simulink model "biplex_core_plan"  (Simulink 7.6)
settings: Solver=ode45  StartTime=0.0  StopTime=10.0  RelTol=1e-3
libraries: xbsIndex_r4 x121, monroe_library x13
settings Model: Creator=Ryan  LastModifiedBy=Ryan

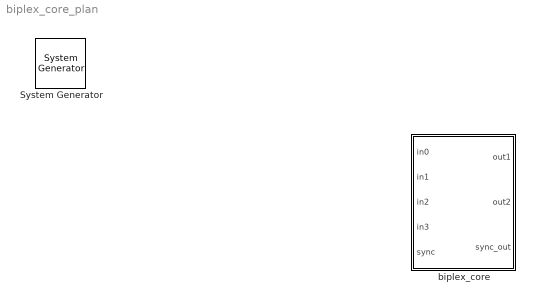
== system biplex_core_plan ==
  " System Generator" : xbsIndex_r4/ System Generator  Tag=genX  SystemSampleTime=-1  xilinxfamily=Virtex6  part=xc6vsx315t  speed=-3  package=ff1156  synthesis_tool=XST  clock_wrapper=Clock Enables  directory=./netlist  testbench=off  simulink_period=1  sysclk_period=10  dcm_input_clock_period=10  incr_netlist=off  trim_vbits=Everywhere in SubSystem  dbl_ovrd=According to Block Masks  core_generation=According to Block Masks  run_coregen=off  deprecated_control=off  eval_field=0  block_type=sysgen
  biplex_core : Subsystem
  wires:
  ? -> biplex_core/5(sync)

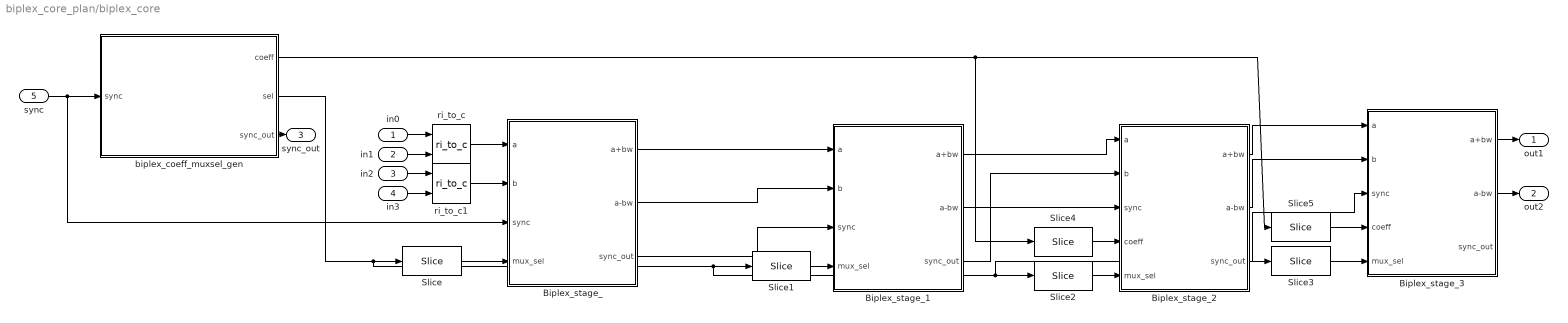
== system biplex_core_plan/biplex_core ==
  in0 : Inport
  in1 : Inport  Port=2
  in2 : Inport  Port=3
  in3 : Inport  Port=4
  sync : Inport  Port=5
  Biplex_stage_ : Subsystem  mask{FFTSize=4, FFTStage=1, input_bit_width=18, coeff_bit_width=18, output_bit_width=18, delays_bram=1, bram_latency=2, shift=0, delay_arr=[0,1,0]}
      mask prompts: FFTSize "FFT Size"; FFTStage "FFT Stage"; input_bit_width "Input Bit Width"; coeff_bit_width "Coefficient Bit Width"; output_bit_width "Output Bit Width"; delays_bram "Delays in BRAM"; bram_latency "BRAM latency"; shift "Downshift in this stage? (0 or 1)"; delay_arr "In-Stage Delay Array"
      mask init:
      | config.source=str2func('biplex_stage_n_draw');
      | config.toplevel=gcb;
      | config.debug=0;
      | config.depend={'biplex_stage_n_draw.m'};
      | xBlock(config,{FFTSize, FFTStage, input_bit_width, coeff_bit_width, output_bit_width, delays_bram, bram_latency, shift, delay_arr});
  Biplex_stage_1 : Subsystem  mask{FFTSize=4, FFTStage=2, input_bit_width=18, coeff_bit_width=18, output_bit_width=18, delays_bram=1, bram_latency=2, shift=0, delay_arr=[0,1,0]}
      mask prompts: FFTSize "FFT Size"; FFTStage "FFT Stage"; input_bit_width "Input Bit Width"; coeff_bit_width "Coefficient Bit Width"; output_bit_width "Output Bit Width"; delays_bram "Delays in BRAM"; bram_latency "BRAM latency"; shift "Downshift in this stage? (0 or 1)"; delay_arr "In-Stage Delay Array"
      mask init: same as biplex_core_plan/biplex_core/Biplex_stage_
  Biplex_stage_2 : Subsystem  mask{FFTSize=4, FFTStage=3, input_bit_width=18, coeff_bit_width=18, output_bit_width=18, delays_bram=1, bram_latency=2, shift=0, delay_arr=[0,1,0]}
      mask prompts: FFTSize "FFT Size"; FFTStage "FFT Stage"; input_bit_width "Input Bit Width"; coeff_bit_width "Coefficient Bit Width"; output_bit_width "Output Bit Width"; delays_bram "Delays in BRAM"; bram_latency "BRAM latency"; shift "Downshift in this stage? (0 or 1)"; delay_arr "In-Stage Delay Array"
      mask init: same as biplex_core_plan/biplex_core/Biplex_stage_
  Biplex_stage_3 : Subsystem  mask{FFTSize=4, FFTStage=4, input_bit_width=18, coeff_bit_width=18, output_bit_width=18, delays_bram=1, bram_latency=2, shift=0, delay_arr=[0,1,0]}
      mask prompts: FFTSize "FFT Size"; FFTStage "FFT Stage"; input_bit_width "Input Bit Width"; coeff_bit_width "Coefficient Bit Width"; output_bit_width "Output Bit Width"; delays_bram "Delays in BRAM"; bram_latency "BRAM latency"; shift "Downshift in this stage? (0 or 1)"; delay_arr "In-Stage Delay Array"
      mask init: same as biplex_core_plan/biplex_core/Biplex_stage_
  Slice : xbsIndex_r4/Slice  nbits=1  boolean_output=on  mode=Upper Bit Location + Width  bit1=0  base1=MSB of Input  bit0=0  base0=LSB of Input  dbl_ovrd=off  block_type=slice
  Slice1 : xbsIndex_r4/Slice  nbits=1  boolean_output=on  mode=Upper Bit Location + Width  bit1=-1  base1=MSB of Input  bit0=0  base0=LSB of Input  dbl_ovrd=off  block_type=slice
  Slice2 : xbsIndex_r4/Slice  nbits=1  boolean_output=on  mode=Upper Bit Location + Width  bit1=-2  base1=MSB of Input  bit0=0  base0=LSB of Input  dbl_ovrd=off  block_type=slice
  Slice3 : xbsIndex_r4/Slice  nbits=1  boolean_output=on  mode=Upper Bit Location + Width  bit1=-3  base1=MSB of Input  bit0=0  base0=LSB of Input  dbl_ovrd=off  block_type=slice
  Slice4 : xbsIndex_r4/Slice  nbits=36  boolean_output=off  mode=Upper Bit Location + Width  bit1=0  base1=MSB of Input  bit0=0  base0=LSB of Input  dbl_ovrd=off  block_type=slice
  Slice5 : xbsIndex_r4/Slice  nbits=36  boolean_output=off  mode=Upper Bit Location + Width  bit1=-36  base1=MSB of Input  bit0=0  base0=LSB of Input  dbl_ovrd=off  block_type=slice
  biplex_coeff_muxsel_gen : Subsystem  mask{FFTSize=4, bit_width=18, register_coeffs=0, optional_delay_arr=[[1,0,1]; [1,1,1];  [1,1,1];  [1,1,1]], stage_delay_arr=[3,6,6,6]}
      mask prompts: FFTSize "FFT Size"; bit_width "Coefficient Bit Width"; register_coeffs "Register Coeffs?"; optional_delay_arr "In-Stage Delay Array"; stage_delay_arr "Mandatory Stage Delay Array"
      mask init:
      | config.source=str2func('biplex_coeff_muxsel_gen_draw');
      | config.toplevel=gcb;
      | config.debug=0;
      | config.depend={'biplex_coeff_muxsel_gen_draw.m'};
      | xBlock(config,{FFTSize, bit_width, register_coeffs, optional_delay_arr, stage_delay_arr});
  ri_to_c : monroe_library/ri_to_c  SystemSampleTime=-1
  ri_to_c1 : monroe_library/ri_to_c  SystemSampleTime=-1
  out1 : Outport
  out2 : Outport  Port=2
  sync_out : Outport  Port=3
  wires:
  ri_to_c/1 -> Biplex_stage_/1(a)
  ri_to_c1/1 -> Biplex_stage_/2(b)
  Biplex_stage_/3(sync_out) -> Biplex_stage_1/3(sync)
  Biplex_stage_/2(a-bw) -> Biplex_stage_1/2(b)
  Biplex_stage_/1(a+bw) -> Biplex_stage_1/1(a)
  Biplex_stage_1/1(a+bw) -> Biplex_stage_2/1(a)
  Biplex_stage_1/2(a-bw) -> Biplex_stage_2/2(b)
  Biplex_stage_1/3(sync_out) -> Biplex_stage_2/3(sync)
  Biplex_stage_2/1(a+bw) -> Biplex_stage_3/1(a)
  Biplex_stage_2/2(a-bw) -> Biplex_stage_3/2(b)
  Biplex_stage_2/3(sync_out) -> Biplex_stage_3/3(sync)
  biplex_coeff_muxsel_gen/2(sel) -> Slice/1, Slice1/1, Slice2/1, Slice3/1
  Slice/1 -> Biplex_stage_/4(mux_sel)
  Slice2/1 -> Biplex_stage_2/5(mux_sel)
  Slice1/1 -> Biplex_stage_1/4(mux_sel)
  Slice3/1 -> Biplex_stage_3/5(mux_sel)
  sync/1 -> biplex_coeff_muxsel_gen/1(sync), Biplex_stage_/3(sync)
  Slice5/1 -> Biplex_stage_3/4(coeff)
  biplex_coeff_muxsel_gen/1(coeff) -> Slice5/1, Slice4/1
  Slice4/1 -> Biplex_stage_2/4(coeff)
  in0/1 -> ri_to_c/1
  biplex_coeff_muxsel_gen/3(sync_out) -> sync_out/1
  Biplex_stage_3/1(a+bw) -> out1/1
  in1/1 -> ri_to_c/2
  in2/1 -> ri_to_c1/1
  in3/1 -> ri_to_c1/2
  Biplex_stage_3/2(a-bw) -> out2/1

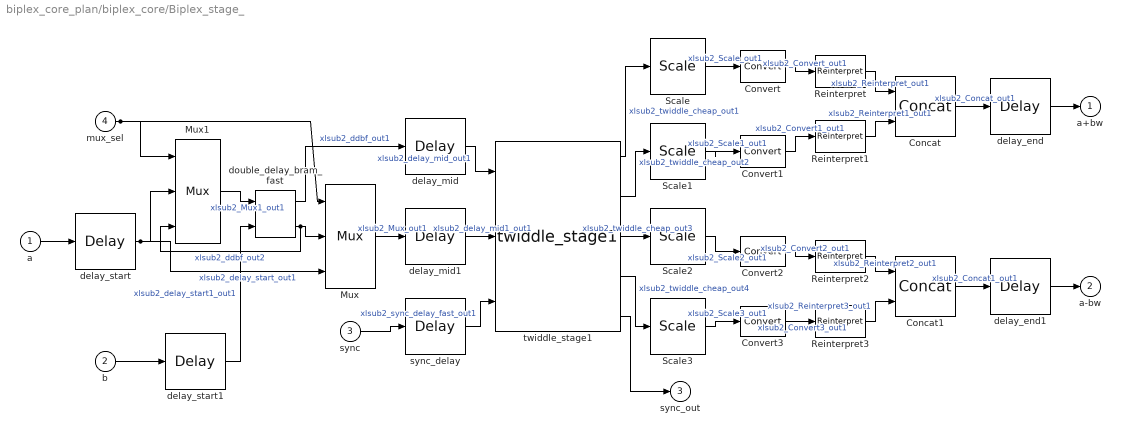
== system biplex_core_plan/biplex_core/Biplex_stage_ ==
  a : Inport
  b : Inport  Port=2
  sync : Inport  Port=3
  mux_sel : Inport  Port=4
  Concat : xbsIndex_r4/Concat  num_inputs=2  dbl_ovrd=off  block_type=concat
  Concat1 : xbsIndex_r4/Concat  num_inputs=2  dbl_ovrd=off  block_type=concat
  Convert{,1..3} (4 alike) : xbsIndex_r4/Convert  arith_type="Signed  (2's comp)"  n_bits=18  bin_pt=17  quantization=Truncate  overflow=Wrap  en=off  latency=0  dbl_ovrd=off  pipeline=off  block_type=convert
  Mux : xbsIndex_r4/Mux  inputs=2  en=off  latency=0  precision=Full  arith_type="Signed  (2's comp)"  n_bits=8  bin_pt=2  quantization=Truncate  overflow=Wrap  dbl_ovrd=off  block_type=mux
  Mux1 : xbsIndex_r4/Mux  inputs=2  en=off  latency=0  precision=Full  arith_type="Signed  (2's comp)"  n_bits=8  bin_pt=2  quantization=Truncate  overflow=Wrap  dbl_ovrd=off  block_type=mux
  Reinterpret{,1..3} (4 alike) : xbsIndex_r4/Reinterpret  force_arith_type=off  arith_type=Unsigned  force_bin_pt=off  bin_pt=0  block_type=reinterpret
      settings: infoedit="Changes signal type without altering the binary representation.   You can changed the signal between signed and unsigned, and relocate the binary point.<br><br>Hardware notes: In hardware this block costs nothing.<br><br>Example:  Suppose the input is 6 bits wide, signed, with 2 fractional bits, and the output is forced to unsigned with 0 fractional bits.  Then an input of -2.0 (1110.00 in binary 2's complement) becomes an output of 56 (111000 in binary)."
  Scale{,1..3} (4 alike) : xbsIndex_r4/Scale  scale_factor=-0  dbl_ovrd=off  block_type=scale
  delay_end : xbsIndex_r4/Delay  en=off  latency=0  dbl_ovrd=off  reg_retiming=off  block_type=delay
  delay_end1 : xbsIndex_r4/Delay  en=off  latency=0  dbl_ovrd=off  reg_retiming=off  block_type=delay
  delay_mid : xbsIndex_r4/Delay  en=off  latency=2  dbl_ovrd=off  reg_retiming=off  block_type=delay
  delay_mid1 : xbsIndex_r4/Delay  en=off  latency=1  dbl_ovrd=off  reg_retiming=off  block_type=delay
  delay_start : xbsIndex_r4/Delay  en=off  latency=0  dbl_ovrd=off  reg_retiming=off  block_type=delay
  delay_start1 : xbsIndex_r4/Delay  en=off  latency=0  dbl_ovrd=off  reg_retiming=off  block_type=delay
  double_delay_bram_fast : monroe_library/double_delay_bram_fast  SystemSampleTime=-1  delay_len=8  bram_latency=2
  sync_delay : xbsIndex_r4/Delay  en=off  latency=8  dbl_ovrd=off  reg_retiming=off  block_type=delay
  twiddle_stage1 : monroe_library/twiddle_stage1  SystemSampleTime=-1  input_bit_width=18
  a+bw : Outport
  a-bw : Outport  Port=2
  sync_out : Outport  Port=3
  wires:
  mux_sel/1 -> Mux1/1, Mux/1
  double_delay_bram_fast/2 -> Mux1/3, Mux/2  "xlsub2_ddbf_out2"
  delay_start/1 -> Mux1/2, Mux/3  "xlsub2_delay_start_out1"
  twiddle_stage1/5 -> sync_out/1
  twiddle_stage1/4 -> Scale3/1  "xlsub2_twiddle_cheap_out4"
  twiddle_stage1/3 -> Scale2/1  "xlsub2_twiddle_cheap_out3"
  twiddle_stage1/2 -> Scale1/1  "xlsub2_twiddle_cheap_out2"
  twiddle_stage1/1 -> Scale/1  "xlsub2_twiddle_cheap_out1"
  sync_delay/1 -> twiddle_stage1/3  "xlsub2_sync_delay_fast_out1"
  delay_mid1/1 -> twiddle_stage1/2  "xlsub2_delay_mid1_out1"
  delay_mid/1 -> twiddle_stage1/1  "xlsub2_delay_mid_out1"
  sync/1 -> sync_delay/1
  delay_start1/1 -> double_delay_bram_fast/2  "xlsub2_delay_start1_out1"
  b/1 -> delay_start1/1
  a/1 -> delay_start/1
  Mux/1 -> delay_mid1/1  "xlsub2_Mux_out1"
  double_delay_bram_fast/1 -> delay_mid/1  "xlsub2_ddbf_out1"
  delay_end1/1 -> a-bw/1
  Concat1/1 -> delay_end1/1  "xlsub2_Concat1_out1"
  delay_end/1 -> a+bw/1
  Concat/1 -> delay_end/1  "xlsub2_Concat_out1"
  Mux1/1 -> double_delay_bram_fast/1  "xlsub2_Mux1_out1"
  Scale3/1 -> Convert3/1  "xlsub2_Scale3_out1"
  Scale2/1 -> Convert2/1  "xlsub2_Scale2_out1"
  Scale1/1 -> Convert1/1  "xlsub2_Scale1_out1"
  Scale/1 -> Convert/1  "xlsub2_Scale_out1"
  Reinterpret3/1 -> Concat1/2  "xlsub2_Reinterpret3_out1"
  Convert3/1 -> Reinterpret3/1  "xlsub2_Convert3_out1"
  Reinterpret2/1 -> Concat1/1  "xlsub2_Reinterpret2_out1"
  Convert2/1 -> Reinterpret2/1  "xlsub2_Convert2_out1"
  Reinterpret1/1 -> Concat/2  "xlsub2_Reinterpret1_out1"
  Convert1/1 -> Reinterpret1/1  "xlsub2_Convert1_out1"
  Reinterpret/1 -> Concat/1  "xlsub2_Reinterpret_out1"
  Convert/1 -> Reinterpret/1  "xlsub2_Convert_out1"

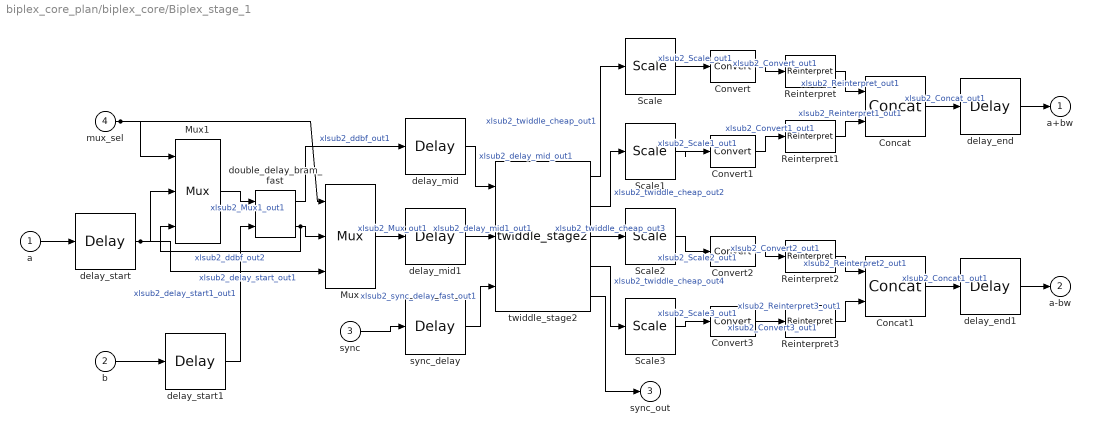
== system biplex_core_plan/biplex_core/Biplex_stage_1 ==
  a : Inport
  b : Inport  Port=2
  sync : Inport  Port=3
  mux_sel : Inport  Port=4
  Concat : xbsIndex_r4/Concat  num_inputs=2  dbl_ovrd=off  block_type=concat
  Concat1 : xbsIndex_r4/Concat  num_inputs=2  dbl_ovrd=off  block_type=concat
  Convert{,1..3} (4 alike) : xbsIndex_r4/Convert  arith_type="Signed  (2's comp)"  n_bits=18  bin_pt=17  quantization=Truncate  overflow=Wrap  en=off  latency=0  dbl_ovrd=off  pipeline=off  block_type=convert
  Mux : xbsIndex_r4/Mux  inputs=2  en=off  latency=0  precision=Full  arith_type="Signed  (2's comp)"  n_bits=8  bin_pt=2  quantization=Truncate  overflow=Wrap  dbl_ovrd=off  block_type=mux
  Mux1 : xbsIndex_r4/Mux  inputs=2  en=off  latency=0  precision=Full  arith_type="Signed  (2's comp)"  n_bits=8  bin_pt=2  quantization=Truncate  overflow=Wrap  dbl_ovrd=off  block_type=mux
  Reinterpret{,1..3} (4 alike) : xbsIndex_r4/Reinterpret  force_arith_type=off  arith_type=Unsigned  force_bin_pt=off  bin_pt=0  block_type=reinterpret
      settings: infoedit="Changes signal type without altering the binary representation.   You can changed the signal between signed and unsigned, and relocate the binary point.<br><br>Hardware notes: In hardware this block costs nothing.<br><br>Example:  Suppose the input is 6 bits wide, signed, with 2 fractional bits, and the output is forced to unsigned with 0 fractional bits.  Then an input of -2.0 (1110.00 in binary 2's complement) becomes an output of 56 (111000 in binary)."
  Scale{,1..3} (4 alike) : xbsIndex_r4/Scale  scale_factor=-0  dbl_ovrd=off  block_type=scale
  delay_end : xbsIndex_r4/Delay  en=off  latency=0  dbl_ovrd=off  reg_retiming=off  block_type=delay
  delay_end1 : xbsIndex_r4/Delay  en=off  latency=0  dbl_ovrd=off  reg_retiming=off  block_type=delay
  delay_mid : xbsIndex_r4/Delay  en=off  latency=2  dbl_ovrd=off  reg_retiming=off  block_type=delay
  delay_mid1 : xbsIndex_r4/Delay  en=off  latency=1  dbl_ovrd=off  reg_retiming=off  block_type=delay
  delay_start : xbsIndex_r4/Delay  en=off  latency=0  dbl_ovrd=off  reg_retiming=off  block_type=delay
  delay_start1 : xbsIndex_r4/Delay  en=off  latency=0  dbl_ovrd=off  reg_retiming=off  block_type=delay
  double_delay_bram_fast : monroe_library/double_delay_bram_fast  SystemSampleTime=-1  delay_len=4  bram_latency=2
  sync_delay : xbsIndex_r4/Delay  en=off  latency=4  dbl_ovrd=off  reg_retiming=off  block_type=delay
  twiddle_stage2 : monroe_library/twiddle_stage2  SystemSampleTime=-1  FFTSize=4  input_bit_width=18
  a+bw : Outport
  a-bw : Outport  Port=2
  sync_out : Outport  Port=3
  wires:
  mux_sel/1 -> Mux1/1, Mux/1
  double_delay_bram_fast/2 -> Mux1/3, Mux/2  "xlsub2_ddbf_out2"
  delay_start/1 -> Mux1/2, Mux/3  "xlsub2_delay_start_out1"
  twiddle_stage2/5 -> sync_out/1
  twiddle_stage2/4 -> Scale3/1  "xlsub2_twiddle_cheap_out4"
  twiddle_stage2/3 -> Scale2/1  "xlsub2_twiddle_cheap_out3"
  twiddle_stage2/2 -> Scale1/1  "xlsub2_twiddle_cheap_out2"
  twiddle_stage2/1 -> Scale/1  "xlsub2_twiddle_cheap_out1"
  sync_delay/1 -> twiddle_stage2/3  "xlsub2_sync_delay_fast_out1"
  delay_mid1/1 -> twiddle_stage2/2  "xlsub2_delay_mid1_out1"
  delay_mid/1 -> twiddle_stage2/1  "xlsub2_delay_mid_out1"
  sync/1 -> sync_delay/1
  delay_start1/1 -> double_delay_bram_fast/2  "xlsub2_delay_start1_out1"
  b/1 -> delay_start1/1
  a/1 -> delay_start/1
  Mux/1 -> delay_mid1/1  "xlsub2_Mux_out1"
  double_delay_bram_fast/1 -> delay_mid/1  "xlsub2_ddbf_out1"
  delay_end1/1 -> a-bw/1
  Concat1/1 -> delay_end1/1  "xlsub2_Concat1_out1"
  delay_end/1 -> a+bw/1
  Concat/1 -> delay_end/1  "xlsub2_Concat_out1"
  Mux1/1 -> double_delay_bram_fast/1  "xlsub2_Mux1_out1"
  Scale3/1 -> Convert3/1  "xlsub2_Scale3_out1"
  Scale2/1 -> Convert2/1  "xlsub2_Scale2_out1"
  Scale1/1 -> Convert1/1  "xlsub2_Scale1_out1"
  Scale/1 -> Convert/1  "xlsub2_Scale_out1"
  Reinterpret3/1 -> Concat1/2  "xlsub2_Reinterpret3_out1"
  Convert3/1 -> Reinterpret3/1  "xlsub2_Convert3_out1"
  Reinterpret2/1 -> Concat1/1  "xlsub2_Reinterpret2_out1"
  Convert2/1 -> Reinterpret2/1  "xlsub2_Convert2_out1"
  Reinterpret1/1 -> Concat/2  "xlsub2_Reinterpret1_out1"
  Convert1/1 -> Reinterpret1/1  "xlsub2_Convert1_out1"
  Reinterpret/1 -> Concat/1  "xlsub2_Reinterpret_out1"
  Convert/1 -> Reinterpret/1  "xlsub2_Convert_out1"

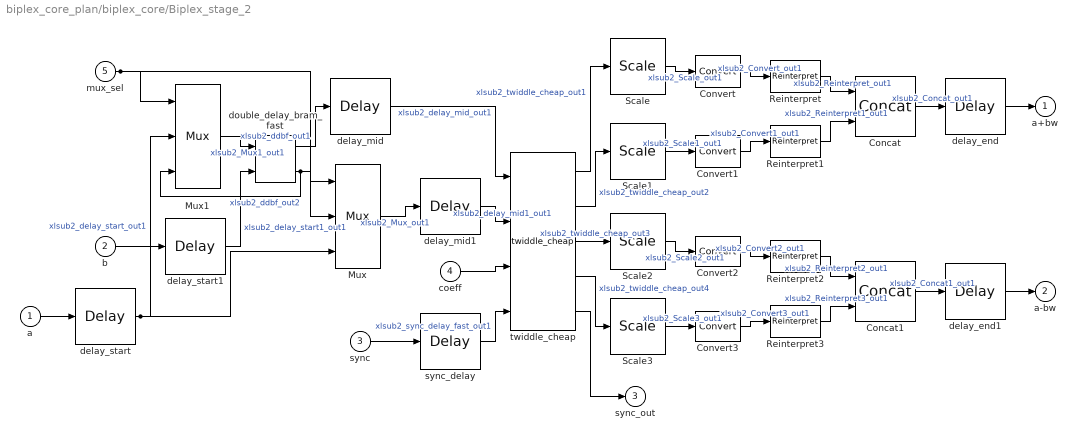
== system biplex_core_plan/biplex_core/Biplex_stage_2 ==
  a : Inport
  b : Inport  Port=2
  sync : Inport  Port=3
  coeff : Inport  Port=4
  mux_sel : Inport  Port=5
  Concat : xbsIndex_r4/Concat  num_inputs=2  dbl_ovrd=off  block_type=concat
  Concat1 : xbsIndex_r4/Concat  num_inputs=2  dbl_ovrd=off  block_type=concat
  Convert{,1..3} (4 alike) : xbsIndex_r4/Convert  arith_type="Signed  (2's comp)"  n_bits=18  bin_pt=17  quantization=Truncate  overflow=Wrap  en=off  latency=0  dbl_ovrd=off  pipeline=off  block_type=convert
  Mux : xbsIndex_r4/Mux  inputs=2  en=off  latency=0  precision=Full  arith_type="Signed  (2's comp)"  n_bits=8  bin_pt=2  quantization=Truncate  overflow=Wrap  dbl_ovrd=off  block_type=mux
  Mux1 : xbsIndex_r4/Mux  inputs=2  en=off  latency=0  precision=Full  arith_type="Signed  (2's comp)"  n_bits=8  bin_pt=2  quantization=Truncate  overflow=Wrap  dbl_ovrd=off  block_type=mux
  Reinterpret{,1..3} (4 alike) : xbsIndex_r4/Reinterpret  force_arith_type=off  arith_type=Unsigned  force_bin_pt=off  bin_pt=0  block_type=reinterpret
      settings: infoedit="Changes signal type without altering the binary representation.   You can changed the signal between signed and unsigned, and relocate the binary point.<br><br>Hardware notes: In hardware this block costs nothing.<br><br>Example:  Suppose the input is 6 bits wide, signed, with 2 fractional bits, and the output is forced to unsigned with 0 fractional bits.  Then an input of -2.0 (1110.00 in binary 2's complement) becomes an output of 56 (111000 in binary)."
  Scale{,1..3} (4 alike) : xbsIndex_r4/Scale  scale_factor=-0  dbl_ovrd=off  block_type=scale
  delay_end : xbsIndex_r4/Delay  en=off  latency=0  dbl_ovrd=off  reg_retiming=off  block_type=delay
  delay_end1 : xbsIndex_r4/Delay  en=off  latency=0  dbl_ovrd=off  reg_retiming=off  block_type=delay
  delay_mid : xbsIndex_r4/Delay  en=off  latency=2  dbl_ovrd=off  reg_retiming=off  block_type=delay
  delay_mid1 : xbsIndex_r4/Delay  en=off  latency=1  dbl_ovrd=off  reg_retiming=off  block_type=delay
  delay_start : xbsIndex_r4/Delay  en=off  latency=0  dbl_ovrd=off  reg_retiming=off  block_type=delay
  delay_start1 : xbsIndex_r4/Delay  en=off  latency=0  dbl_ovrd=off  reg_retiming=off  block_type=delay
  double_delay_bram_fast : monroe_library/double_delay_bram_fast  SystemSampleTime=-1  delay_len=2  bram_latency=2
  sync_delay : xbsIndex_r4/Delay  en=off  latency=2  dbl_ovrd=off  reg_retiming=off  block_type=delay
  twiddle_cheap : monroe_library/twiddle_cheap  SystemSampleTime=-1  a_n_bits=18  a_bin_pt=17  b_n_bits=18  b_bin_pt=17  w_n_bits=18  w_bin_pt=17  a_delay=0
  a+bw : Outport
  a-bw : Outport  Port=2
  sync_out : Outport  Port=3
  wires:
  mux_sel/1 -> Mux1/1, Mux/1
  double_delay_bram_fast/2 -> Mux1/3, Mux/2  "xlsub2_ddbf_out2"
  delay_start/1 -> Mux1/2, Mux/3  "xlsub2_delay_start_out1"
  twiddle_cheap/5 -> sync_out/1
  twiddle_cheap/4 -> Scale3/1  "xlsub2_twiddle_cheap_out4"
  twiddle_cheap/3 -> Scale2/1  "xlsub2_twiddle_cheap_out3"
  twiddle_cheap/2 -> Scale1/1  "xlsub2_twiddle_cheap_out2"
  twiddle_cheap/1 -> Scale/1  "xlsub2_twiddle_cheap_out1"
  sync_delay/1 -> twiddle_cheap/4  "xlsub2_sync_delay_fast_out1"
  coeff/1 -> twiddle_cheap/3
  delay_mid1/1 -> twiddle_cheap/2  "xlsub2_delay_mid1_out1"
  delay_mid/1 -> twiddle_cheap/1  "xlsub2_delay_mid_out1"
  sync/1 -> sync_delay/1
  delay_start1/1 -> double_delay_bram_fast/2  "xlsub2_delay_start1_out1"
  b/1 -> delay_start1/1
  a/1 -> delay_start/1
  Mux/1 -> delay_mid1/1  "xlsub2_Mux_out1"
  double_delay_bram_fast/1 -> delay_mid/1  "xlsub2_ddbf_out1"
  delay_end1/1 -> a-bw/1
  Concat1/1 -> delay_end1/1  "xlsub2_Concat1_out1"
  delay_end/1 -> a+bw/1
  Concat/1 -> delay_end/1  "xlsub2_Concat_out1"
  Mux1/1 -> double_delay_bram_fast/1  "xlsub2_Mux1_out1"
  Scale3/1 -> Convert3/1  "xlsub2_Scale3_out1"
  Scale2/1 -> Convert2/1  "xlsub2_Scale2_out1"
  Scale1/1 -> Convert1/1  "xlsub2_Scale1_out1"
  Scale/1 -> Convert/1  "xlsub2_Scale_out1"
  Reinterpret3/1 -> Concat1/2  "xlsub2_Reinterpret3_out1"
  Convert3/1 -> Reinterpret3/1  "xlsub2_Convert3_out1"
  Reinterpret2/1 -> Concat1/1  "xlsub2_Reinterpret2_out1"
  Convert2/1 -> Reinterpret2/1  "xlsub2_Convert2_out1"
  Reinterpret1/1 -> Concat/2  "xlsub2_Reinterpret1_out1"
  Convert1/1 -> Reinterpret1/1  "xlsub2_Convert1_out1"
  Reinterpret/1 -> Concat/1  "xlsub2_Reinterpret_out1"
  Convert/1 -> Reinterpret/1  "xlsub2_Convert_out1"

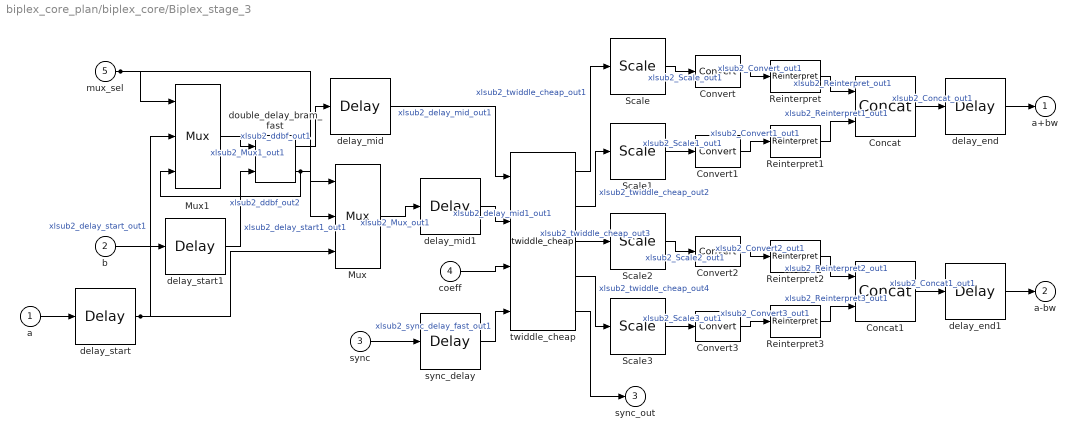
== system biplex_core_plan/biplex_core/Biplex_stage_3 ==
  a : Inport
  b : Inport  Port=2
  sync : Inport  Port=3
  coeff : Inport  Port=4
  mux_sel : Inport  Port=5
  Concat : xbsIndex_r4/Concat  num_inputs=2  dbl_ovrd=off  block_type=concat
  Concat1 : xbsIndex_r4/Concat  num_inputs=2  dbl_ovrd=off  block_type=concat
  Convert{,1..3} (4 alike) : xbsIndex_r4/Convert  arith_type="Signed  (2's comp)"  n_bits=18  bin_pt=17  quantization=Truncate  overflow=Wrap  en=off  latency=0  dbl_ovrd=off  pipeline=off  block_type=convert
  Mux : xbsIndex_r4/Mux  inputs=2  en=off  latency=0  precision=Full  arith_type="Signed  (2's comp)"  n_bits=8  bin_pt=2  quantization=Truncate  overflow=Wrap  dbl_ovrd=off  block_type=mux
  Mux1 : xbsIndex_r4/Mux  inputs=2  en=off  latency=0  precision=Full  arith_type="Signed  (2's comp)"  n_bits=8  bin_pt=2  quantization=Truncate  overflow=Wrap  dbl_ovrd=off  block_type=mux
  Reinterpret{,1..3} (4 alike) : xbsIndex_r4/Reinterpret  force_arith_type=off  arith_type=Unsigned  force_bin_pt=off  bin_pt=0  block_type=reinterpret
      settings: infoedit="Changes signal type without altering the binary representation.   You can changed the signal between signed and unsigned, and relocate the binary point.<br><br>Hardware notes: In hardware this block costs nothing.<br><br>Example:  Suppose the input is 6 bits wide, signed, with 2 fractional bits, and the output is forced to unsigned with 0 fractional bits.  Then an input of -2.0 (1110.00 in binary 2's complement) becomes an output of 56 (111000 in binary)."
  Scale{,1..3} (4 alike) : xbsIndex_r4/Scale  scale_factor=-0  dbl_ovrd=off  block_type=scale
  delay_end : xbsIndex_r4/Delay  en=off  latency=0  dbl_ovrd=off  reg_retiming=off  block_type=delay
  delay_end1 : xbsIndex_r4/Delay  en=off  latency=0  dbl_ovrd=off  reg_retiming=off  block_type=delay
  delay_mid : xbsIndex_r4/Delay  en=off  latency=2  dbl_ovrd=off  reg_retiming=off  block_type=delay
  delay_mid1 : xbsIndex_r4/Delay  en=off  latency=1  dbl_ovrd=off  reg_retiming=off  block_type=delay
  delay_start : xbsIndex_r4/Delay  en=off  latency=0  dbl_ovrd=off  reg_retiming=off  block_type=delay
  delay_start1 : xbsIndex_r4/Delay  en=off  latency=0  dbl_ovrd=off  reg_retiming=off  block_type=delay
  double_delay_bram_fast : monroe_library/double_delay_bram_fast  SystemSampleTime=-1  delay_len=1  bram_latency=2
  sync_delay : xbsIndex_r4/Delay  en=off  latency=1  dbl_ovrd=off  reg_retiming=off  block_type=delay
  twiddle_cheap : monroe_library/twiddle_cheap  SystemSampleTime=-1  a_n_bits=18  a_bin_pt=17  b_n_bits=18  b_bin_pt=17  w_n_bits=18  w_bin_pt=17  a_delay=0
  a+bw : Outport
  a-bw : Outport  Port=2
  sync_out : Outport  Port=3
  wires:
  mux_sel/1 -> Mux1/1, Mux/1
  double_delay_bram_fast/2 -> Mux1/3, Mux/2  "xlsub2_ddbf_out2"
  delay_start/1 -> Mux1/2, Mux/3  "xlsub2_delay_start_out1"
  twiddle_cheap/5 -> sync_out/1
  twiddle_cheap/4 -> Scale3/1  "xlsub2_twiddle_cheap_out4"
  twiddle_cheap/3 -> Scale2/1  "xlsub2_twiddle_cheap_out3"
  twiddle_cheap/2 -> Scale1/1  "xlsub2_twiddle_cheap_out2"
  twiddle_cheap/1 -> Scale/1  "xlsub2_twiddle_cheap_out1"
  sync_delay/1 -> twiddle_cheap/4  "xlsub2_sync_delay_fast_out1"
  coeff/1 -> twiddle_cheap/3
  delay_mid1/1 -> twiddle_cheap/2  "xlsub2_delay_mid1_out1"
  delay_mid/1 -> twiddle_cheap/1  "xlsub2_delay_mid_out1"
  sync/1 -> sync_delay/1
  delay_start1/1 -> double_delay_bram_fast/2  "xlsub2_delay_start1_out1"
  b/1 -> delay_start1/1
  a/1 -> delay_start/1
  Mux/1 -> delay_mid1/1  "xlsub2_Mux_out1"
  double_delay_bram_fast/1 -> delay_mid/1  "xlsub2_ddbf_out1"
  delay_end1/1 -> a-bw/1
  Concat1/1 -> delay_end1/1  "xlsub2_Concat1_out1"
  delay_end/1 -> a+bw/1
  Concat/1 -> delay_end/1  "xlsub2_Concat_out1"
  Mux1/1 -> double_delay_bram_fast/1  "xlsub2_Mux1_out1"
  Scale3/1 -> Convert3/1  "xlsub2_Scale3_out1"
  Scale2/1 -> Convert2/1  "xlsub2_Scale2_out1"
  Scale1/1 -> Convert1/1  "xlsub2_Scale1_out1"
  Scale/1 -> Convert/1  "xlsub2_Scale_out1"
  Reinterpret3/1 -> Concat1/2  "xlsub2_Reinterpret3_out1"
  Convert3/1 -> Reinterpret3/1  "xlsub2_Convert3_out1"
  Reinterpret2/1 -> Concat1/1  "xlsub2_Reinterpret2_out1"
  Convert2/1 -> Reinterpret2/1  "xlsub2_Convert2_out1"
  Reinterpret1/1 -> Concat/2  "xlsub2_Reinterpret1_out1"
  Convert1/1 -> Reinterpret1/1  "xlsub2_Convert1_out1"
  Reinterpret/1 -> Concat/1  "xlsub2_Reinterpret_out1"
  Convert/1 -> Reinterpret/1  "xlsub2_Convert_out1"

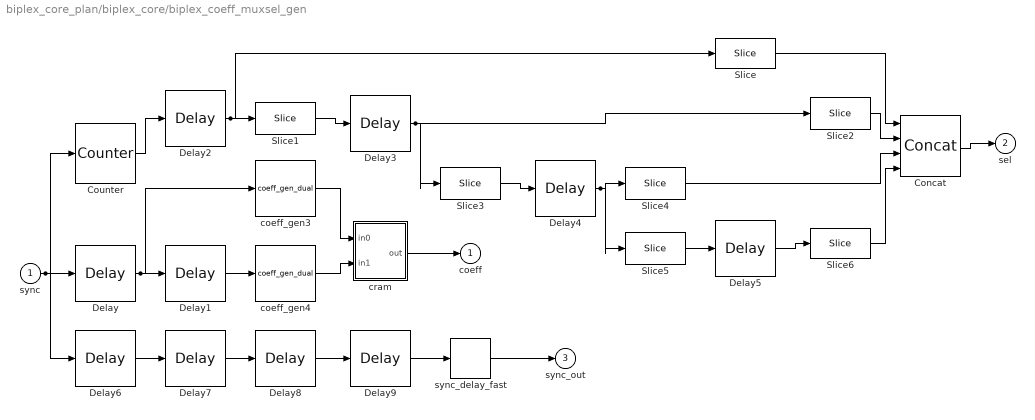
== system biplex_core_plan/biplex_core/biplex_coeff_muxsel_gen ==
  sync : Inport
  Concat : xbsIndex_r4/Concat  num_inputs=4  dbl_ovrd=off  block_type=concat
  Counter : xbsIndex_r4/Counter  cnt_type=Free Running  cnt_to=Inf  operation=Up  start_count=0  cnt_by_val=1  arith_type=Unsigned  n_bits=3  bin_pt=0  load_pin=off  rst=on  en=off  explicit_period=on  period=1  dbl_ovrd=off  use_behavioral_HDL=off  implementation=Fabric  block_type=counter
  Delay : xbsIndex_r4/Delay  en=off  latency=16  dbl_ovrd=off  reg_retiming=off  block_type=delay
  Delay1 : xbsIndex_r4/Delay  en=off  latency=9  dbl_ovrd=off  reg_retiming=off  block_type=delay
  Delay{2,6..9} (5 alike) : xbsIndex_r4/Delay  en=off  latency=1  dbl_ovrd=off  reg_retiming=off  block_type=delay
  Delay3 : xbsIndex_r4/Delay  en=off  latency=5  dbl_ovrd=off  reg_retiming=off  block_type=delay
  Delay4 : xbsIndex_r4/Delay  en=off  latency=9  dbl_ovrd=off  reg_retiming=off  block_type=delay
  Delay5 : xbsIndex_r4/Delay  en=off  latency=9  dbl_ovrd=off  reg_retiming=off  block_type=delay
  Slice{,1..6} (7 alike) : xbsIndex_r4/Slice  nbits=1  boolean_output=off  mode=Upper Bit Location + Width  bit1=0  base1=MSB of Input  bit0=0  base0=MSB of Input  dbl_ovrd=off  block_type=slice
  coeff_gen3 : monroe_library/coeff_gen_dual  SystemSampleTime=-1  coeff=[0 -1 -0.707106781186547 -0.707106781186548 1 6.12323399573677e-017 0.707106781186548 -0.707106781186547]  bit_width=18  register_output=0
  coeff_gen4 : monroe_library/coeff_gen_dual  SystemSampleTime=-1  coeff=[0 -1 -0.707106781186547 -0.707106781186548 -0.38268343236509 -0.923879532511287 -0.923879532511287 -0.38268343236509 1 6.12323399573677e-017 0.707106781186548 -0.707106781186547 0.923879532511287 -0.38268343236509 0.38268343236509 -0.923879532511287]  bit_width=18  register_output=0
  cram : Subsystem
  sync_delay_fast : monroe_library/sync_delay_fast  SystemSampleTime=-1  delay_len=85
  coeff : Outport
  sel : Outport  Port=2
  sync_out : Outport  Port=3
  wires:
  sync/1 -> Delay6/1, Counter/1, Delay/1
  Delay/1 -> Delay1/1, coeff_gen3/1
  Delay2/1 -> Slice1/1, Slice/1
  Delay3/1 -> Slice3/1, Slice2/1
  Delay4/1 -> Slice5/1, Slice4/1
  sync_delay_fast/1 -> sync_out/1
  Delay9/1 -> sync_delay_fast/1
  Delay8/1 -> Delay9/1
  Delay7/1 -> Delay8/1
  Delay6/1 -> Delay7/1
  Concat/1 -> sel/1
  Slice6/1 -> Concat/4
  Slice4/1 -> Concat/3
  Slice2/1 -> Concat/2
  Slice/1 -> Concat/1
  Delay5/1 -> Slice6/1
  Slice5/1 -> Delay5/1
  Slice3/1 -> Delay4/1
  Slice1/1 -> Delay3/1
  Counter/1 -> Delay2/1
  cram/1(out) -> coeff/1
  coeff_gen4/1 -> cram/2(in1)
  coeff_gen3/1 -> cram/1(in0)
  Delay1/1 -> coeff_gen4/1

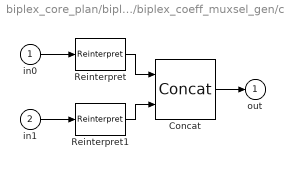
== system biplex_core_plan/biplex_core/biplex_coeff_muxsel_gen/cram ==
  in0 : Inport
  in1 : Inport  Port=2
  Concat : xbsIndex_r4/Concat  num_inputs=2  dbl_ovrd=off  block_type=concat
  Reinterpret : xbsIndex_r4/Reinterpret  force_arith_type=on  arith_type=Unsigned  force_bin_pt=on  bin_pt=0  block_type=reinterpret
      settings: infoedit="Changes signal type without altering the binary representation.   You can changed the signal between signed and unsigned, and relocate the binary point.<br><br>Hardware notes: In hardware this block costs nothing.<br><br>Example:  Suppose the input is 6 bits wide, signed, with 2 fractional bits, and the output is forced to unsigned with 0 fractional bits.  Then an input of -2.0 (1110.00 in binary 2's complement) becomes an output of 56 (111000 in binary)."
  Reinterpret1 : xbsIndex_r4/Reinterpret  force_arith_type=on  arith_type=Unsigned  force_bin_pt=on  bin_pt=0  block_type=reinterpret
      settings: infoedit="Changes signal type without altering the binary representation.   You can changed the signal between signed and unsigned, and relocate the binary point.<br><br>Hardware notes: In hardware this block costs nothing.<br><br>Example:  Suppose the input is 6 bits wide, signed, with 2 fractional bits, and the output is forced to unsigned with 0 fractional bits.  Then an input of -2.0 (1110.00 in binary 2's complement) becomes an output of 56 (111000 in binary)."
  out : Outport
  wires:
  Reinterpret1/1 -> Concat/2
  in1/1 -> Reinterpret1/1
  Reinterpret/1 -> Concat/1
  in0/1 -> Reinterpret/1
  Concat/1 -> out/1
